simulink library "lib_controls"  (Simulink 7.9)
settings: Solver=ode45  SolverMode=SingleTasking  StartTime=0.0  StopTime=10.0  RelTol=1e-3
undefined symbols (not defined in the file or in its folder): amb_tmp, cs_charge_deplete_bool, cs_charge_pwr, cs_charge_trq, cs_clt_tmp, cs_decel_fc_off, cs_decel_regen_threshold, cs_dl_assist_trq_threshold, cs_dl_regen_trq_threshold, cs_electric_decel_spd, cs_electric_launch_spd, cs_electric_launch_spd_hi, cs_electric_launch_spd_lo, cs_eng_min_spd, cs_eng_on_soc, cs_fc_init_state, cs_fc_max_pwr_frac, cs_fc_min_pwr_frac, cs_fc_on, cs_fc_pwr_opt, cs_fc_spd_opt, cs_fuzzy_fuel_mode, cs_hi_soc, cs_hi_trq_frac, cs_lo_soc, cs_lo_trq_frac, cs_max_gc_spd, cs_max_pwr, cs_max_pwr_fall_rate, cs_max_pwr_rise_rate, cs_mc_assist_max_frac, cs_mc_assist_min_frac, cs_mc_assist_slope, cs_mc_regen_max_frac, cs_mc_regen_min_frac, cs_mc_regen_slope, cs_mean_eff, cs_mean_eff_bool, cs_min_gc_spd, cs_min_off_time, cs_min_pwr, cs_min_trq_frac, cs_mph_avg_time, cs_off_trq_frac, cs_plot_output, cs_pwr, cs_regen_avg_time, cs_scale_factor, cs_shutoff, cs_soc_range, cs_spd, cs_target_soc, cs_trq_to_soc_factor, cvt_locus_pwr, cvt_locus_spd, cyc_mph, enable_sim_stop_distance, enable_sim_stop_max_spd, enable_sim_stop_speed, enable_sim_stop_time ... (+110)
libraries: lib_controls x124, simulink3 x13, simulink x5, lib_etc x1
(part 10 of 17)

== system lib_controls/series hybrid control stategy  <cs>/pwr req'd from FC to supply pwr req'd at bus (W) ==
  power req'd by bus (W) : Inport
  Constant : Constant  Value=eps
  Constant1 : Constant  Value=eps
  Constant2 : Constant  Value=0
  Constant3 : Constant  Value=0
  Constant4 : Constant  Value=eps
  Relational Operator : RelationalOperator  Operator=>  InputSameDT=on
  Saturation : Saturate  UpperLimit=max(cs_pwr)  LowerLimit=min(cs_pwr)
  Sum : Sum  SaturateOnIntegerOverflow=on  InputSameDT=on  OutDataTypeStr=Inherit: Same as first input
  Sum1 : Sum  SaturateOnIntegerOverflow=on  InputSameDT=on  OutDataTypeStr=Inherit: Same as first input
  Sum2 : Sum  SaturateOnIntegerOverflow=on  InputSameDT=on  OutDataTypeStr=Inherit: Same as first input
  Switch : Switch  Threshold=eps  SaturateOnIntegerOverflow=on  InputSameDT=on
  est. efficiency : Product  Inputs=*/  SaturateOnIntegerOverflow=on  RndMeth=Zero  InputSameDT=on  OutDataTypeStr=Inherit: Same as first input
  est. desired spd (rad/s) : Lookup  InputValues=cs_pwr  Table=cs_spd  SaturateOnIntegerOverflow=on
  est. desired trq (Nm) : Product  Inputs=*/  SaturateOnIntegerOverflow=on  RndMeth=Zero  InputSameDT=on  OutDataTypeStr=Inherit: Same as first input
  est. pwr req'd into generator : Product  Inputs=/*  SaturateOnIntegerOverflow=on  RndMeth=Zero  InputSameDT=on  OutDataTypeStr=Inherit: Same as first input
  generator output power map (W) : Lookup2D  RowIndex=gc_map_spd*gc_spd_scale  ColumnIndex=gc_map_trq*gc_trq_scale  Table=gc_outpwr_map*gc_spd_scale*gc_trq_scale  SaturateOnIntegerOverflow=on  InputSameDT=on
  pwr req'd of FC (W) : Outport
  wires:
  power req'd by bus (W)/1 -> Relational Operator/1, Saturation/1
  Constant2/1 -> Relational Operator/2
  Constant1/1 -> Sum1/1
  Sum1/1 -> est. efficiency/2
  generator output power map (W)/1 -> est. efficiency/1
  Saturation/1 -> Sum1/2, est. pwr req'd into generator/2, est. desired trq (Nm)/1, est. desired spd (rad/s)/1
  est. desired spd (rad/s)/1 -> generator output power map (W)/1, Sum/1
  est. desired trq (Nm)/1 -> generator output power map (W)/2
  Constant/1 -> Sum/2
  Sum/1 -> est. desired trq (Nm)/2
  Constant3/1 -> Switch/3
  Relational Operator/1 -> Switch/2
  Switch/1 -> pwr req'd of FC (W)/1
  est. pwr req'd into generator/1 -> Switch/1
  est. efficiency/1 -> Sum2/1
  Sum2/1 -> est. pwr req'd into generator/1
  Constant4/1 -> Sum2/2

== system lib_controls/series hybrid control stategy  <cs>/thermostat ==

== system lib_controls/user contributed engine on (balanced parallel hybrid)/Block NOTES ==
  note: this user-contributed model came from Serve Ploumen-Research Engineer in Energy Management
      |  at Ford Forschungszentrum Aachen GmbH (Ford Research Centre Aachen)
      | The following is from the email:
      | For integrated Starter/generator equipped vehicles, we found it important to make the activation of
      | engine start-stop dependent on thetime needed for the engine-warmup (or catalyst warmup if you like)
      |  and also dependent in the SOC of the energy storage device. Furthermore we found
      | it important to delay the engine shut-down after the vehicle has come to a stop after a braking period.
      |
      | Therefore we implemented these functionality in the control strategy of Advisor's parallel hybrid model.

== system lib_controls/<vc> conv/clutch control/Block NOTES ==
  note: This clutch control block determines the clutch state given the req'd clutch output torque
      | and speed (labelled as gearbox input torque and speed), and the gear number history.
      |                           conditions                                                                       clutch state
      | gear is being shifted OR (trq <~ 0 AND (engine is                                     1 == disengaged
      | clutched to avoid compression braking OR spd < idle))
      |
      | (trq >~ 0) AND (spd < launch speed) AND clutch                                       2 == slipping
      | was not engaged during previous time step
      |
      | neither of above sets of conditions are met                                          3 == engaged

== system lib_controls/<vc> conv/clutch control/gearbox speed estimator ==
  gb_spd_in_r if no gear change : Inport
  Block NOTES : Subsystem
      mask Display: disp('Block\nNOTES')
  Constant : Constant  Value=eps
  Constant1 : Constant  Value=0
  Constant2 : Constant
  Constant3 : Constant  Value=0.11
  Gain : Gain  Gain=0.447  SaturateOnIntegerOverflow=on  OutDataTypeStr=Inherit: Same as input  ParamDataTypeStr=Inherit: Same as input
  Logical : Logic
  Memory : Memory  X0=cyc_mph(1,2)*0.447/wh_radius*fd_ratio*gb_ratio(gb_num_init)
  Memory1 : Memory  X0=1
  Product : Product  Inputs=**/  SaturateOnIntegerOverflow=on  RndMeth=Zero  InputSameDT=on  OutDataTypeStr=Inherit: Same as first input
  Relational : RelationalOperator  Operator=>  InputSameDT=on
  Relational1 : RelationalOperator  Operator=<=  InputSameDT=on
  Sum : Sum  SaturateOnIntegerOverflow=on  InputSameDT=on  OutDataTypeStr=Inherit: Same as first input
  Sum1 : Sum  Inputs=-+  SaturateOnIntegerOverflow=on  InputSameDT=on  OutDataTypeStr=Inherit: Same as first input
  Switch : Switch  Threshold=eps  SaturateOnIntegerOverflow=on  InputSameDT=on
  Switch1 : Switch  Threshold=eps  SaturateOnIntegerOverflow=on  InputSameDT=on
  dt : Subsystem
  Out1 : Outport
  wires:
  dt/1(Out1) -> Relational1/1
  Logical/1 -> Switch1/2
  Memory1/1 -> Logical/1
  Relational1/1 -> Logical/2
  Constant3/1 -> Relational1/2
  [gb_spd_in_a] -> Product/1
  gb_spd_in_r if no gear change/1 -> Switch1/3
  Switch1/1 -> Out1/1
  Switch/1 -> Memory/1
  Relational/1 -> Memory1/1
  Sum1/1 -> Relational/1
  Constant2/1 -> Relational/2
  [mpha] -> Sum1/1, Gain/1
  [cyc_mph_r] -> Sum1/2
  Constant/1 -> Sum/2
  Memory/1 -> Switch1/1
  Constant1/1 -> Switch/3
  [veh_spd_a_rec] -> Switch/2, Sum/1
  Gain/1 -> Product/2
  Sum/1 -> Product/3
  Product/1 -> Switch/1

== system lib_controls/<vc> conv/engine control/Block NOTES ==
  note: This engine control block determines whether the engine is on, which it is when
      | [(the clutch is slipping or engaged OR idling is allowed) AND the ignition key is on]
      | OR
      | (the transmission is shifting AND the engine was on during the previous time step).
      | The second part involving shifting is to prevent the engine from shutting down
      | for 1 or 2 seconds during shifts.

== system lib_controls/<vc> conv/engine control/key_on ==
  Clock : Clock
  Fcn1 : Fcn  Expr=rem(u[1],period)
  Look-Up Table : Lookup  InputValues=t  Table=y  SaturateOnIntegerOverflow=on
  out_1 : Outport  InitialOutput=0
  wires:
  Fcn1/1 -> Look-Up Table/1
  Clock/1 -> Fcn1/1
  Look-Up Table/1 -> out_1/1

== system lib_controls/<vc> conv/engine control/repeated cycle:  speed required at end of NEXT step ==
  Clock : Clock
  Fcn1 : Fcn  Expr=rem(u[1],period)
  Look-Up Table : Lookup  InputValues=t  Table=y  SaturateOnIntegerOverflow=on
  Memory : Memory  X0=-0.1
  Sum : Sum  Inputs=+-  SaturateOnIntegerOverflow=on  InputSameDT=on  OutDataTypeStr=Inherit: Same as first input
  Sum1 : Sum  SaturateOnIntegerOverflow=on  InputSameDT=on  OutDataTypeStr=Inherit: Same as first input
  out_1 : Outport  InitialOutput=0
  wires:
  Clock/1 -> Sum/1, Memory/1, Fcn1/1
  Memory/1 -> Sum/2
  Sum/1 -> Sum1/2
  Fcn1/1 -> Sum1/1
  Look-Up Table/1 -> out_1/1
  Sum1/1 -> Look-Up Table/1

== system lib_controls/<vc> conv/gearbox  control/Block NOTES ==
  note: This gearbox control block computes the current gear number given the gearbox's
      | req'd output torque and speed and an estimate its efficiency.  Upshifts occur, given a
      | certain engine speed,  when the estimated engine load falls below the upshift curve
      | in engine speed/load space, and downshifts likewise occur when estimated engine
      | load rises above the downshift curve.  Separate upshift and downshift curves are
      | defined for each gear.  An upshift may not be immediately followed by a downshift.
      | If the tires are about to slip, don't upshift unless the engine would be at max. speed.
      | Enforce this rule by setting the load to 1 when the tires are about to slip.

== system lib_controls/<vc> conv/gearbox  control/allow downshift? ==
  prev gearnum : Inport
  Logical Operator : Logic  Operator=NOR
  Memory : Memory  X0=1
  Memory1 : Memory  X0=1
  Relational Operator1 : RelationalOperator  Operator=>  InputSameDT=on
  Relational Operator2 : RelationalOperator  Operator=>  InputSameDT=on
  allow shift : Outport  InitialOutput=0
  wires:
  Relational Operator2/1 -> Logical Operator/2
  Memory1/1 -> Relational Operator2/2
  Memory/1 -> Memory1/1, Relational Operator1/2
  Relational Operator1/1 -> Logical Operator/1
  prev gearnum/1 -> Relational Operator2/1, Memory/1, Relational Operator1/1
  Logical Operator/1 -> allow shift/1

== system lib_controls/<vc> conv/gearbox  control/downshift  command ==
  prev gear number : Inport
  engine load : Inport  Port=2
  engine speed : Inport  Port=3
  Mux : Mux  Inputs=2
  Relational Operator : RelationalOperator  Operator=>  InputSameDT=on
  load fraction : Subsystem  mask(Gear Selector){spd=gb_dnshift_spd, load=gb_dnshift_load}
      mask prompts: spd "Speeds:"; load "Load Fractions:"
      mask help:
      | This block will perform a linear interplation (extrapolation outside of bounds) to determine the shift point load fraction associated with the current gear number and speed.
      |
      | The Speeds parameter should be defined as an array of vectors containing speeds for each gear number.  The Load Fractions parameter should be defined as a array of vectors containing load fractions indexed by the speeds in the Speeds parameter for each gear number.
      mask Help:
      | Reference the base workspace variables - gb_**shift_spd and gb_**shift_load  where ** is either up for upshift conditions or dn for downshift conditions.
      | 
      | Or define the arrays as follows:
      | 
      | {[spd1 spd2 spd3 spd4]; [spd1 spd2 spd3 spd4]; ...}
      | 
      | {[load1 load2 load3 load4]; [load1 load2 load3 load4]; ...}
      | 
      | where each array contains one row for each gear in the gearbox.  Speeds should be defined in rad/s and loads as a decimal fraction.
  command : Outport  InitialOutput=0
  wires:
  Relational Operator/1 -> command/1
  engine speed/1 -> Mux/2
  prev gear number/1 -> Mux/1
  engine load/1 -> Relational Operator/1
  Mux/1 -> load fraction/1(In1)
  load fraction/1(Out1) -> Relational Operator/2

== system lib_controls/<vc> conv/gearbox  control/gearbox speed estimator ==
  gb_spd_in_r if no gear change : Inport
  Block NOTES : Subsystem
      mask Display: disp('Block\nNOTES')
  Constant : Constant  Value=eps
  Constant1 : Constant  Value=0
  Constant2 : Constant
  Constant3 : Constant  Value=0.11
  Gain : Gain  Gain=0.447  SaturateOnIntegerOverflow=on  OutDataTypeStr=Inherit: Same as input  ParamDataTypeStr=Inherit: Same as input
  Logical : Logic
  Memory : Memory  X0=cyc_mph(1,2)*0.447/wh_radius*fd_ratio*gb_ratio(gb_num_init)
  Memory1 : Memory  X0=1
  Product : Product  Inputs=**/  SaturateOnIntegerOverflow=on  RndMeth=Zero  InputSameDT=on  OutDataTypeStr=Inherit: Same as first input
  Relational : RelationalOperator  Operator=>  InputSameDT=on
  Relational1 : RelationalOperator  Operator=<=  InputSameDT=on
  Sum : Sum  SaturateOnIntegerOverflow=on  InputSameDT=on  OutDataTypeStr=Inherit: Same as first input
  Sum1 : Sum  Inputs=-+  SaturateOnIntegerOverflow=on  InputSameDT=on  OutDataTypeStr=Inherit: Same as first input
  Switch : Switch  Threshold=eps  SaturateOnIntegerOverflow=on  InputSameDT=on
  Switch1 : Switch  Threshold=eps  SaturateOnIntegerOverflow=on  InputSameDT=on
  dt : Subsystem
  Out1 : Outport
  wires:
  dt/1(Out1) -> Relational1/1
  Logical/1 -> Switch1/2
  Memory1/1 -> Logical/1
  Relational1/1 -> Logical/2
  Constant3/1 -> Relational1/2
  [gb_spd_in_a] -> Product/1
  gb_spd_in_r if no gear change/1 -> Switch1/3
  Switch1/1 -> Out1/1
  Switch/1 -> Memory/1
  Relational/1 -> Memory1/1
  Sum1/1 -> Relational/1
  Constant2/1 -> Relational/2
  [mpha] -> Sum1/1, Gain/1
  [cyc_mph_r] -> Sum1/2
  Constant/1 -> Sum/2
  Memory/1 -> Switch1/1
  Constant1/1 -> Switch/3
  [veh_spd_a_rec] -> Switch/2, Sum/1
  Gain/1 -> Product/2
  Sum/1 -> Product/3
  Product/1 -> Switch/1

== system lib_controls/<vc> conv/gearbox  control/shifting1 ==
  gear number : Inport
  Constant : Constant  Value=gb_shift_delay-1e-6
  Relational Operator : RelationalOperator  Operator=<  InputSameDT=on
  time since last shift : Subsystem
      mask Display: disp('time since\nlast shift')
  out_1 : Outport  InitialOutput=0
  wires:
  time since last shift/1(out_1) -> Relational Operator/1
  Constant/1 -> Relational Operator/2
  gear number/1 -> time since last shift/1(in_1)
  Relational Operator/1 -> out_1/1

== system lib_controls/<vc> conv/gearbox  control/upshift  command ==
  prev gear number : Inport
  engine load : Inport  Port=2
  engine speed : Inport  Port=3
  Mux : Mux  Inputs=2
  Relational Operator : RelationalOperator  Operator=<  InputSameDT=on
  load fraction : Subsystem  mask(Gear Selector){spd=gb_upshift_spd, load=gb_upshift_load}
      mask prompts: spd "Speeds:"; load "Load Fractions:"
      mask help:
      | This block will perform a linear interplation (extrapolation outside of bounds) to determine the shift point load fraction associated with the current gear number and speed.
      |
      | The Speeds parameter should be defined as an array of vectors containing speeds for each gear number.  The Load Fractions parameter should be defined as a array of vectors containing load fractions indexed by the speeds in the Speeds parameter for each gear number.
      mask Help:
      | Reference the base workspace variables - gb_**shift_spd and gb_**shift_load  where ** is either up for upshift conditions or dn for downshift conditions.
      | 
      | Or define the arrays as follows:
      | 
      | {[spd1 spd2 spd3 spd4]; [spd1 spd2 spd3 spd4]; ...}
      | 
      | {[load1 load2 load3 load4]; [load1 load2 load3 load4]; ...}
      | 
      | where each array contains one row for each gear in the gearbox.  Speeds should be defined in rad/s and loads as a decimal fraction.
  command : Outport  InitialOutput=0
  wires:
  Relational Operator/1 -> command/1
  engine speed/1 -> Mux/2
  Mux/1 -> load fraction/1(In1)
  prev gear number/1 -> Mux/1
  engine load/1 -> Relational Operator/1
  load fraction/1(Out1) -> Relational Operator/2

== system lib_controls/<vc> conv Saber custom/clutch control/Block NOTES ==
  note: This clutch control block determines the clutch state given the req'd clutch output torque
      | and speed (labelled as gearbox input torque and speed), and the gear number history.
      |                           conditions                                                                       clutch state
      | gear is being shifted OR (trq <~ 0 AND (engine is                                     1 == disengaged
      | clutched to avoid compression braking OR spd < idle))
      |
      | (trq >~ 0) AND (spd < launch speed) AND clutch                                       2 == slipping
      | was not engaged during previous time step
      |
      | neither of above sets of conditions are met                                          3 == engaged

== system lib_controls/<vc> conv Saber custom/clutch control/gearbox speed estimator ==
  gb_spd_in_r if no gear change : Inport
  Block NOTES : Subsystem
      mask Display: disp('Block\nNOTES')
  Constant : Constant  Value=eps
  Constant1 : Constant  Value=0
  Constant2 : Constant
  Constant3 : Constant  Value=0.11
  Gain : Gain  Gain=0.447  SaturateOnIntegerOverflow=on  OutDataTypeStr=Inherit: Same as input  ParamDataTypeStr=Inherit: Same as input
  Logical : Logic
  Memory : Memory  X0=cyc_mph(1,2)*0.447/wh_radius*fd_ratio*gb_ratio(gb_num_init)
  Memory1 : Memory  X0=1
  Product : Product  Inputs=**/  SaturateOnIntegerOverflow=on  RndMeth=Zero  InputSameDT=on  OutDataTypeStr=Inherit: Same as first input
  Relational : RelationalOperator  Operator=>  InputSameDT=on
  Relational1 : RelationalOperator  Operator=<=  InputSameDT=on
  Sum : Sum  SaturateOnIntegerOverflow=on  InputSameDT=on  OutDataTypeStr=Inherit: Same as first input
  Sum1 : Sum  Inputs=-+  SaturateOnIntegerOverflow=on  InputSameDT=on  OutDataTypeStr=Inherit: Same as first input
  Switch : Switch  Threshold=eps  SaturateOnIntegerOverflow=on  InputSameDT=on
  Switch1 : Switch  Threshold=eps  SaturateOnIntegerOverflow=on  InputSameDT=on
  dt : Subsystem
  Out1 : Outport
  wires:
  Product/1 -> Switch/1
  Sum/1 -> Product/3
  Gain/1 -> Product/2
  [veh_spd_a_rec] -> Sum/1, Switch/2
  Constant1/1 -> Switch/3
  Memory/1 -> Switch1/1
  Constant/1 -> Sum/2
  [cyc_mph_r] -> Sum1/2
  [mpha] -> Gain/1, Sum1/1
  Constant2/1 -> Relational/2
  Sum1/1 -> Relational/1
  Relational/1 -> Memory1/1
  Switch/1 -> Memory/1
  Switch1/1 -> Out1/1
  gb_spd_in_r if no gear change/1 -> Switch1/3
  [gb_spd_in_a] -> Product/1
  Constant3/1 -> Relational1/2
  Relational1/1 -> Logical/2
  Memory1/1 -> Logical/1
  Logical/1 -> Switch1/2
  dt/1(Out1) -> Relational1/1

== system lib_controls/<vc> conv Saber custom/engine control/Block NOTES ==
  note: This engine control block determines whether the engine is on, which it is when
      | [(the clutch is slipping or engaged OR idling is allowed) AND the ignition key is on]
      | OR
      | (the transmission is shifting AND the engine was on during the previous time step).
      | The second part involving shifting is to prevent the engine from shutting down
      | for 1 or 2 seconds during shifts.

== system lib_controls/<vc> conv Saber custom/engine control/key_on ==
  Clock : Clock
  Fcn1 : Fcn  Expr=rem(u[1],period)
  Look-Up Table : Lookup  InputValues=t  Table=y  SaturateOnIntegerOverflow=on
  out_1 : Outport  InitialOutput=0
  wires:
  Look-Up Table/1 -> out_1/1
  Clock/1 -> Fcn1/1
  Fcn1/1 -> Look-Up Table/1

== system lib_controls/<vc> conv Saber custom/engine control/repeated cycle:  speed required at end of NEXT step ==
  Clock : Clock
  Fcn1 : Fcn  Expr=rem(u[1],period)
  Look-Up Table : Lookup  InputValues=t  Table=y  SaturateOnIntegerOverflow=on
  Memory : Memory  X0=-0.1
  Sum : Sum  Inputs=+-  SaturateOnIntegerOverflow=on  InputSameDT=on  OutDataTypeStr=Inherit: Same as first input
  Sum1 : Sum  SaturateOnIntegerOverflow=on  InputSameDT=on  OutDataTypeStr=Inherit: Same as first input
  out_1 : Outport  InitialOutput=0
  wires:
  Sum1/1 -> Look-Up Table/1
  Look-Up Table/1 -> out_1/1
  Fcn1/1 -> Sum1/1
  Sum/1 -> Sum1/2
  Memory/1 -> Sum/2
  Clock/1 -> Fcn1/1, Memory/1, Sum/1

== system lib_controls/<vc> conv Saber custom/gearbox  control/Block NOTES ==
  note: This gearbox control block computes the current gear number given the gearbox's
      | req'd output torque and speed and an estimate its efficiency.  Upshifts occur, given a
      | certain engine speed,  when the estimated engine load falls below the upshift curve
      | in engine speed/load space, and downshifts likewise occur when estimated engine
      | load rises above the downshift curve.  Separate upshift and downshift curves are
      | defined for each gear.  An upshift may not be immediately followed by a downshift.
      | If the tires are about to slip, don't upshift unless the engine would be at max. speed.
      | Enforce this rule by setting the load to 1 when the tires are about to slip.

== system lib_controls/<vc> conv Saber custom/gearbox  control/accessories (Nm) ==
  T_acc : Outport  InitialOutput=0
  wires:
  [fc_acc_trq_r] -> T_acc/1

== system lib_controls/<vc> conv Saber custom/gearbox  control/allow downshift? ==
  prev gearnum : Inport
  Logical Operator : Logic  Operator=NOR
  Memory : Memory  X0=1
  Memory1 : Memory  X0=1
  Relational Operator1 : RelationalOperator  Operator=>  InputSameDT=on
  Relational Operator2 : RelationalOperator  Operator=>  InputSameDT=on
  allow shift : Outport  InitialOutput=0
  wires:
  Logical Operator/1 -> allow shift/1
  prev gearnum/1 -> Relational Operator1/1, Memory/1, Relational Operator2/1
  Relational Operator1/1 -> Logical Operator/1
  Memory/1 -> Relational Operator1/2, Memory1/1
  Memory1/1 -> Relational Operator2/2
  Relational Operator2/1 -> Logical Operator/2

== system lib_controls/<vc> conv Saber custom/gearbox  control/downshift  command ==
  prev gear number : Inport
  engine load : Inport  Port=2
  engine speed : Inport  Port=3
  Mux : Mux  Inputs=2
  Relational Operator : RelationalOperator  Operator=>  InputSameDT=on
  load fraction : Subsystem  mask(Gear Selector){spd=gb_dnshift_spd, load=gb_dnshift_load}
      mask prompts: spd "Speeds:"; load "Load Fractions:"
      mask help:
      | This block will perform a linear interplation (extrapolation outside of bounds) to determine the shift point load fraction associated with the current gear number and speed.
      |
      | The Speeds parameter should be defined as an array of vectors containing speeds for each gear number.  The Load Fractions parameter should be defined as a array of vectors containing load fractions indexed by the speeds in the Speeds parameter for each gear number.
      mask Help:
      | Reference the base workspace variables - gb_**shift_spd and gb_**shift_load  where ** is either up for upshift conditions or dn for downshift conditions.
      | 
      | Or define the arrays as follows:
      | 
      | {[spd1 spd2 spd3 spd4]; [spd1 spd2 spd3 spd4]; ...}
      | 
      | {[load1 load2 load3 load4]; [load1 load2 load3 load4]; ...}
      | 
      | where each array contains one row for each gear in the gearbox.  Speeds should be defined in rad/s and loads as a decimal fraction.
  command : Outport  InitialOutput=0
  wires:
  load fraction/1(Out1) -> Relational Operator/2
  Mux/1 -> load fraction/1(In1)
  engine load/1 -> Relational Operator/1
  prev gear number/1 -> Mux/1
  engine speed/1 -> Mux/2
  Relational Operator/1 -> command/1

== system lib_controls/<vc> conv Saber custom/gearbox  control/gearbox speed estimator ==
  gb_spd_in_r if no gear change : Inport
  Block NOTES : Subsystem
      mask Display: disp('Block\nNOTES')
  Constant : Constant  Value=eps
  Constant1 : Constant  Value=0
  Constant2 : Constant
  Constant3 : Constant  Value=0.11
  Gain : Gain  Gain=0.447  SaturateOnIntegerOverflow=on  OutDataTypeStr=Inherit: Same as input  ParamDataTypeStr=Inherit: Same as input
  Logical : Logic
  Memory : Memory  X0=cyc_mph(1,2)*0.447/wh_radius*fd_ratio*gb_ratio(gb_num_init)
  Memory1 : Memory  X0=1
  Product : Product  Inputs=**/  SaturateOnIntegerOverflow=on  RndMeth=Zero  InputSameDT=on  OutDataTypeStr=Inherit: Same as first input
  Relational : RelationalOperator  Operator=>  InputSameDT=on
  Relational1 : RelationalOperator  Operator=<=  InputSameDT=on
  Sum : Sum  SaturateOnIntegerOverflow=on  InputSameDT=on  OutDataTypeStr=Inherit: Same as first input
  Sum1 : Sum  Inputs=-+  SaturateOnIntegerOverflow=on  InputSameDT=on  OutDataTypeStr=Inherit: Same as first input
  Switch : Switch  Threshold=eps  SaturateOnIntegerOverflow=on  InputSameDT=on
  Switch1 : Switch  Threshold=eps  SaturateOnIntegerOverflow=on  InputSameDT=on
  dt : Subsystem
  Out1 : Outport
  wires:
  Product/1 -> Switch/1
  Sum/1 -> Product/3
  Gain/1 -> Product/2
  [veh_spd_a_rec] -> Sum/1, Switch/2
  Constant1/1 -> Switch/3
  Memory/1 -> Switch1/1
  Constant/1 -> Sum/2
  [cyc_mph_r] -> Sum1/2
  [mpha] -> Gain/1, Sum1/1
  Constant2/1 -> Relational/2
  Sum1/1 -> Relational/1
  Relational/1 -> Memory1/1
  Switch/1 -> Memory/1
  Switch1/1 -> Out1/1
  gb_spd_in_r if no gear change/1 -> Switch1/3
  [gb_spd_in_a] -> Product/1
  Constant3/1 -> Relational1/2
  Relational1/1 -> Logical/2
  Memory1/1 -> Logical/1
  Logical/1 -> Switch1/2
  dt/1(Out1) -> Relational1/1

== system lib_controls/<vc> conv Saber custom/gearbox  control/shifting1 ==
  gear number : Inport
  Constant : Constant  Value=gb_shift_delay-1e-6
  Relational Operator : RelationalOperator  Operator=<  InputSameDT=on
  time since last shift : Subsystem
      mask Display: disp('time since\nlast shift')
  out_1 : Outport  InitialOutput=0
  wires:
  Relational Operator/1 -> out_1/1
  gear number/1 -> time since last shift/1(in_1)
  Constant/1 -> Relational Operator/2
  time since last shift/1(out_1) -> Relational Operator/1

== system lib_controls/<vc> conv Saber custom/gearbox  control/upshift  command ==
  prev gear number : Inport
  engine load : Inport  Port=2
  engine speed : Inport  Port=3
  Mux : Mux  Inputs=2
  Relational Operator : RelationalOperator  Operator=<  InputSameDT=on
  load fraction : Subsystem  mask(Gear Selector){spd=gb_upshift_spd, load=gb_upshift_load}
      mask prompts: spd "Speeds:"; load "Load Fractions:"
      mask help:
      | This block will perform a linear interplation (extrapolation outside of bounds) to determine the shift point load fraction associated with the current gear number and speed.
      |
      | The Speeds parameter should be defined as an array of vectors containing speeds for each gear number.  The Load Fractions parameter should be defined as a array of vectors containing load fractions indexed by the speeds in the Speeds parameter for each gear number.
      mask Help:
      | Reference the base workspace variables - gb_**shift_spd and gb_**shift_load  where ** is either up for upshift conditions or dn for downshift conditions.
      | 
      | Or define the arrays as follows:
      | 
      | {[spd1 spd2 spd3 spd4]; [spd1 spd2 spd3 spd4]; ...}
      | 
      | {[load1 load2 load3 load4]; [load1 load2 load3 load4]; ...}
      | 
      | where each array contains one row for each gear in the gearbox.  Speeds should be defined in rad/s and loads as a decimal fraction.
  command : Outport  InitialOutput=0
  wires:
  load fraction/1(Out1) -> Relational Operator/2
  engine load/1 -> Relational Operator/1
  prev gear number/1 -> Mux/1
  Mux/1 -> load fraction/1(In1)
  engine speed/1 -> Mux/2
  Relational Operator/1 -> command/1

== system lib_controls/<vc> conv auto/engine control/Block NOTES ==
  note: This engine control block determines whether the engine is on, which it is when
      | [(the clutch is slipping or engaged OR idling is allowed) AND the ignition key is on]
      | OR
      | (the transmission is shifting AND the engine was on during the previous time step).
      | The second part involving shifting is to prevent the engine from shutting down
      | for 1 or 2 seconds during shifts.

== system lib_controls/<vc> conv auto/engine control/key_on ==
  Clock : Clock
  Fcn1 : Fcn  Expr=rem(u[1],period)
  Look-Up Table : Lookup  InputValues=t  Table=y  SaturateOnIntegerOverflow=on
  out_1 : Outport  InitialOutput=0
  wires:
  Look-Up Table/1 -> out_1/1
  Clock/1 -> Fcn1/1
  Fcn1/1 -> Look-Up Table/1

== system lib_controls/<vc> conv auto/engine control/repeated cycle:  speed required at end of NEXT step ==
  Clock : Clock
  Fcn1 : Fcn  Expr=rem(u[1],period)
  Look-Up Table : Lookup  InputValues=t  Table=y  SaturateOnIntegerOverflow=on
  Memory : Memory  X0=-0.1
  Sum : Sum  Inputs=+-  SaturateOnIntegerOverflow=on  InputSameDT=on  OutDataTypeStr=Inherit: Same as first input
  Sum1 : Sum  SaturateOnIntegerOverflow=on  InputSameDT=on  OutDataTypeStr=Inherit: Same as first input
  out_1 : Outport  InitialOutput=0
  wires:
  Clock/1 -> Sum/1, Memory/1, Fcn1/1
  Memory/1 -> Sum/2
  Sum/1 -> Sum1/2
  Fcn1/1 -> Sum1/1
  Look-Up Table/1 -> out_1/1
  Sum1/1 -> Look-Up Table/1

== system lib_controls/<vc> conv auto/gearbox control for use w/ AT/Block NOTES ==
  note: This gearbox control block computes the current gear number given the gearbox's
      | req'd output torque and speed and an estimate its efficiency.  Upshifts occur, given a
      | certain engine speed,  when the estimated engine load falls below the upshift curve
      | in engine speed/load space, and downshifts likewise occur when estimated engine
      | load rises above the downshift curve.  Separate upshift and downshift curves are
      | defined for each gear.  An upshift may not be immediately followed by a downshift.
      | If the tires are about to slip, don't upshift unless the engine would be at max. speed.
      | Enforce this rule by setting the load to 1 when the tires are about to slip.
  note: Lock-up of the HTC occurs when it is supposed to for the current gear, AND
      | the transmission isn't shifting, AND
      | the lockup wouldn't precipitate an immediate downshift.

== system lib_controls/<vc> conv auto/gearbox control for use w/ AT/allow downshift? ==
  prev gearnum : Inport
  Logical Operator : Logic  Operator=NOR
  Memory : Memory  X0=1
  Memory1 : Memory  X0=1
  Relational Operator1 : RelationalOperator  Operator=>  InputSameDT=on
  Relational Operator2 : RelationalOperator  Operator=>  InputSameDT=on
  allow shift : Outport  InitialOutput=0
  wires:
  Relational Operator2/1 -> Logical Operator/2
  Memory1/1 -> Relational Operator2/2
  Memory/1 -> Memory1/1, Relational Operator1/2
  Relational Operator1/1 -> Logical Operator/1
  prev gearnum/1 -> Relational Operator2/1, Memory/1, Relational Operator1/1
  Logical Operator/1 -> allow shift/1

== system lib_controls/<vc> conv auto/gearbox control for use w/ AT/downshift  command ==
  prev gear number : Inport
  engine load : Inport  Port=2
  engine speed : Inport  Port=3
  Mux : Mux  Inputs=2
  Relational Operator : RelationalOperator  Operator=>  InputSameDT=on
  load fraction : Subsystem  mask(Gear Selector){spd=gb_dnshift_spd, load=gb_dnshift_load}
      mask prompts: spd "Speeds:"; load "Load Fractions:"
      mask help:
      | This block will perform a linear interplation (extrapolation outside of bounds) to determine the shift point load fraction associated with the current gear number and speed.
      |
      | The Speeds parameter should be defined as an array of vectors containing speeds for each gear number.  The Load Fractions parameter should be defined as a array of vectors containing load fractions indexed by the speeds in the Speeds parameter for each gear number.
      mask Help:
      | Reference the base workspace variables - gb_**shift_spd and gb_**shift_load  where ** is either up for upshift conditions or dn for downshift conditions.
      | 
      | Or define the arrays as follows:
      | 
      | {[spd1 spd2 spd3 spd4]; [spd1 spd2 spd3 spd4]; ...}
      | 
      | {[load1 load2 load3 load4]; [load1 load2 load3 load4]; ...}
      | 
      | where each array contains one row for each gear in the gearbox.  Speeds should be defined in rad/s and loads as a decimal fraction.
  command : Outport  InitialOutput=0
  wires:
  load fraction/1(Out1) -> Relational Operator/2
  Mux/1 -> load fraction/1(In1)
  engine load/1 -> Relational Operator/1
  prev gear number/1 -> Mux/1
  engine speed/1 -> Mux/2
  Relational Operator/1 -> command/1

== system lib_controls/<vc> conv auto/gearbox control for use w/ AT/downshift  command1 ==
  prev gear number : Inport
  engine load : Inport  Port=2
  engine speed : Inport  Port=3
  Mux : Mux  Inputs=2
  Relational Operator : RelationalOperator  Operator=>  InputSameDT=on
  load fraction : Subsystem  mask(Gear Selector){spd=gb_dnshift_spd, load=gb_dnshift_load}
      mask prompts: spd "Speeds:"; load "Load Fractions:"
      mask help:
      | This block will perform a linear interplation (extrapolation outside of bounds) to determine the shift point load fraction associated with the current gear number and speed.
      |
      | The Speeds parameter should be defined as an array of vectors containing speeds for each gear number.  The Load Fractions parameter should be defined as a array of vectors containing load fractions indexed by the speeds in the Speeds parameter for each gear number.
      mask Help:
      | Reference the base workspace variables - gb_**shift_spd and gb_**shift_load  where ** is either up for upshift conditions or dn for downshift conditions.
      | 
      | Or define the arrays as follows:
      | 
      | {[spd1 spd2 spd3 spd4]; [spd1 spd2 spd3 spd4]; ...}
      | 
      | {[load1 load2 load3 load4]; [load1 load2 load3 load4]; ...}
      | 
      | where each array contains one row for each gear in the gearbox.  Speeds should be defined in rad/s and loads as a decimal fraction.
  command : Outport  InitialOutput=0
  wires:
  Relational Operator/1 -> command/1
  prev gear number/1 -> Mux/1
  engine load/1 -> Relational Operator/1
  Mux/1 -> load fraction/1(In1)
  load fraction/1(Out1) -> Relational Operator/2
  engine speed/1 -> Mux/2

== system lib_controls/<vc> conv auto/gearbox control for use w/ AT/est. engine trq and spd ==
  prev gear number : Inport
  " prev eta_gb" : Inport  Port=2
  gb_trq_out_r : Inport  Port=3
  gb_spd_out_r : Inport  Port=4
  Block NOTES : Subsystem
      mask Display: disp('Block\nNOTES')
  Constant2 : Constant  Value=[1 1]
  Constant5 : Constant  Value=0
  Demux : Demux  Outputs=2
  K_adv : Subsystem
  Logical Operator : Logic
  Logical Operator1 : Logic  Operator=NOT  Inputs=1
  Memory : Memory
  Mux1 : Mux  Inputs=2
  Mux2 : Mux  Inputs=2
  Relational Operator1 : RelationalOperator  Operator=>  InputSameDT=on
  SR Look-Up Table SR=wout/win : Lookup  InputValues=htc_k_adv  Table=htc_sr  SaturateOnIntegerOverflow=on
  Saturation1 : Saturate  UpperLimit=1  LowerLimit=0.7
  Saturation2 : Saturate  UpperLimit=inf  LowerLimit=0
  Switch : Switch  Threshold=eps  SaturateOnIntegerOverflow=on  InputSameDT=on
  TR Look-Up Table TR=Tout/Tin : Lookup  InputValues=htc_k_adv  Table=htc_tr  SaturateOnIntegerOverflow=on
  TR,SR : Mux  Inputs=2
  est eng trq : Sum  SaturateOnIntegerOverflow=on  InputSameDT=on  OutDataTypeStr=Inherit: Same as first input
  gear ratio1 : Lookup  InputValues=[1:length(gb_ratio)]  Table=gb_ratio  SaturateOnIntegerOverflow=on
  ~eng trq and spd : Product  Inputs=*/  SaturateOnIntegerOverflow=on  RndMeth=Zero  InputSameDT=on  OutDataTypeStr=Inherit: Same as first input
  ~gb_spd_in_r : Product  SaturateOnIntegerOverflow=on  RndMeth=Zero  InputSameDT=on  OutDataTypeStr=Inherit: Same as first input
  ~gb_trq_in_r : Product  Inputs=//*  SaturateOnIntegerOverflow=on  RndMeth=Zero  InputSameDT=on  OutDataTypeStr=Inherit: Same as first input
  est eng trq (Nm) : Outport
  est eng spd (rad/s) : Outport  Port=2
  gb_spd_in_est (rad/s)1 : Outport  Port=3
  wires:
  gb_trq_out_r/1 -> ~gb_trq_in_r/3
  gb_spd_out_r/1 -> ~gb_spd_in_r/2
  gear ratio1/1 -> ~gb_trq_in_r/1, ~gb_spd_in_r/1
  TR,SR/1 -> Switch/1
  Constant2/1 -> Switch/3
  Switch/1 -> ~eng trq and spd/2
  " prev eta_gb"/1 -> Saturation1/1
  Saturation1/1 -> ~gb_trq_in_r/2
  Demux/2 -> Saturation2/1
  Saturation2/1 -> est eng spd (rad/s)/1
  Constant5/1 -> Relational Operator1/2
  Relational Operator1/1 -> Logical Operator/1
  prev gear number/1 -> gear ratio1/1
  Demux/1 -> est eng trq (Nm)/1
  Memory/1 -> Logical Operator1/1
  Logical Operator1/1 -> Logical Operator/2
  Logical Operator/1 -> Switch/2
  [locked_up] -> Memory/1
  Mux1/1 -> ~eng trq and spd/1
  ~eng trq and spd/1 -> Demux/1
  Mux2/1 -> K_adv/1("Req'd output trq and spd (Nm), (rad/s)")
  K_adv/1(K_adv) -> TR Look-Up Table TR=Tout/Tin/1, SR Look-Up Table SR=wout/win/1
  TR Look-Up Table TR=Tout/Tin/1 -> TR,SR/1
  SR Look-Up Table SR=wout/win/1 -> TR,SR/2
  [acc_mech_trq_est] -> est eng trq/2
  ~gb_spd_in_r/1 -> Mux1/2, gb_spd_in_est (rad/s)1/1, Mux2/2
  ~gb_trq_in_r/1 -> est eng trq/1
  est eng trq/1 -> Mux2/1, Relational Operator1/1, Mux1/1

== system lib_controls/<vc> conv auto/gearbox control for use w/ AT/est. engine trq and spd assuming lockup ==
  new gear number : Inport
  " prev eta_gb" : Inport  Port=2
  gb_trq_out_r : Inport  Port=3
  gb_spd_in_est : Inport  Port=4
  Block NOTES : Subsystem
      mask Display: disp('Block\nNOTES')
  Memory : Memory  X0=gb_ratio(1)
  Saturation1 : Saturate  UpperLimit=1  LowerLimit=0.7
  Saturation2 : Saturate  UpperLimit=inf  LowerLimit=0
  est eng trq : Sum  SaturateOnIntegerOverflow=on  InputSameDT=on  OutDataTypeStr=Inherit: Same as first input
  gear ratio1 : Lookup  InputValues=[1:length(gb_ratio)]  Table=gb_ratio  SaturateOnIntegerOverflow=on
  ~gb_spd_in_r : Product  Inputs=*/*  SaturateOnIntegerOverflow=on  RndMeth=Zero  InputSameDT=on  OutDataTypeStr=Inherit: Same as first input
  ~gb_trq_in_r : Product  Inputs=//*  SaturateOnIntegerOverflow=on  RndMeth=Zero  InputSameDT=on  OutDataTypeStr=Inherit: Same as first input
  est eng trq (Nm) : Outport
  est eng spd (rad/s) : Outport  Port=2
  wires:
  Saturation1/1 -> ~gb_trq_in_r/2
  " prev eta_gb"/1 -> Saturation1/1
  gear ratio1/1 -> ~gb_trq_in_r/1, ~gb_spd_in_r/1, Memory/1
  gb_trq_out_r/1 -> ~gb_trq_in_r/3
  new gear number/1 -> gear ratio1/1
  Saturation2/1 -> est eng spd (rad/s)/1
  Memory/1 -> ~gb_spd_in_r/2
  gb_spd_in_est/1 -> ~gb_spd_in_r/3
  [acc_mech_trq_est] -> est eng trq/2
  ~gb_trq_in_r/1 -> est eng trq/1
  est eng trq/1 -> est eng trq (Nm)/1
  ~gb_spd_in_r/1 -> Saturation2/1

== system lib_controls/<vc> conv auto/gearbox control for use w/ AT/shifting1 ==
  gear number : Inport
  Constant : Constant  Value=gb_shift_delay-1e-6
  Relational Operator : RelationalOperator  Operator=<  InputSameDT=on
  time since last shift : Subsystem
      mask Display: disp('time since\nlast shift')
  out_1 : Outport  InitialOutput=0
  wires:
  time since last shift/1(out_1) -> Relational Operator/1
  Constant/1 -> Relational Operator/2
  gear number/1 -> time since last shift/1(in_1)
  Relational Operator/1 -> out_1/1

== system lib_controls/<vc> conv auto/gearbox control for use w/ AT/upshift  command ==
  prev gear number : Inport
  engine load : Inport  Port=2
  engine speed : Inport  Port=3
  Mux : Mux  Inputs=2
  Relational Operator : RelationalOperator  Operator=<  InputSameDT=on
  load fraction : Subsystem  mask(Gear Selector){spd=gb_upshift_spd, load=gb_upshift_load}
      mask prompts: spd "Speeds:"; load "Load Fractions:"
      mask help:
      | This block will perform a linear interplation (extrapolation outside of bounds) to determine the shift point load fraction associated with the current gear number and speed.
      |
      | The Speeds parameter should be defined as an array of vectors containing speeds for each gear number.  The Load Fractions parameter should be defined as a array of vectors containing load fractions indexed by the speeds in the Speeds parameter for each gear number.
      mask Help:
      | Reference the base workspace variables - gb_**shift_spd and gb_**shift_load  where ** is either up for upshift conditions or dn for downshift conditions.
      | 
      | Or define the arrays as follows:
      | 
      | {[spd1 spd2 spd3 spd4]; [spd1 spd2 spd3 spd4]; ...}
      | 
      | {[load1 load2 load3 load4]; [load1 load2 load3 load4]; ...}
      | 
      | where each array contains one row for each gear in the gearbox.  Speeds should be defined in rad/s and loads as a decimal fraction.
  command : Outport  InitialOutput=0
  wires:
  load fraction/1(Out1) -> Relational Operator/2
  engine load/1 -> Relational Operator/1
  prev gear number/1 -> Mux/1
  Mux/1 -> load fraction/1(In1)
  engine speed/1 -> Mux/2
  Relational Operator/1 -> command/1

== system lib_controls/<vc> conv auto Saber custom/engine control/Block NOTES ==
  note: This engine control block determines whether the engine is on, which it is when
      | [(the clutch is slipping or engaged OR idling is allowed) AND the ignition key is on]
      | OR
      | (the transmission is shifting AND the engine was on during the previous time step).
      | The second part involving shifting is to prevent the engine from shutting down
      | for 1 or 2 seconds during shifts.

== system lib_controls/<vc> conv auto Saber custom/engine control/key_on ==
  Clock : Clock
  Fcn1 : Fcn  Expr=rem(u[1],period)
  Look-Up Table : Lookup  InputValues=t  Table=y  SaturateOnIntegerOverflow=on
  out_1 : Outport  InitialOutput=0
  wires:
  Fcn1/1 -> Look-Up Table/1
  Clock/1 -> Fcn1/1
  Look-Up Table/1 -> out_1/1

== system lib_controls/<vc> conv auto Saber custom/engine control/repeated cycle:  speed required at end of NEXT step ==
  Clock : Clock
  Fcn1 : Fcn  Expr=rem(u[1],period)
  Look-Up Table : Lookup  InputValues=t  Table=y  SaturateOnIntegerOverflow=on
  Memory : Memory  X0=-0.1
  Sum : Sum  Inputs=+-  SaturateOnIntegerOverflow=on  InputSameDT=on  OutDataTypeStr=Inherit: Same as first input
  Sum1 : Sum  SaturateOnIntegerOverflow=on  InputSameDT=on  OutDataTypeStr=Inherit: Same as first input
  out_1 : Outport  InitialOutput=0
  wires:
  Sum1/1 -> Look-Up Table/1
  Look-Up Table/1 -> out_1/1
  Fcn1/1 -> Sum1/1
  Sum/1 -> Sum1/2
  Memory/1 -> Sum/2
  Clock/1 -> Fcn1/1, Memory/1, Sum/1

== system lib_controls/<vc> conv auto Saber custom/gearbox control for use w/ AT/Block NOTES ==
  note: Lock-up of the HTC occurs when it is supposed to for the current gear, AND
      | the transmission isn't shifting, AND
      | the lockup wouldn't precipitate an immediate downshift.
  note: This gearbox control block computes the current gear number given the gearbox's
      | req'd output torque and speed and an estimate its efficiency.  Upshifts occur, given a
      | certain engine speed,  when the estimated engine load falls below the upshift curve
      | in engine speed/load space, and downshifts likewise occur when estimated engine
      | load rises above the downshift curve.  Separate upshift and downshift curves are
      | defined for each gear.  An upshift may not be immediately followed by a downshift.
      | If the tires are about to slip, don't upshift unless the engine would be at max. speed.
      | Enforce this rule by setting the load to 1 when the tires are about to slip.

== system lib_controls/<vc> conv auto Saber custom/gearbox control for use w/ AT/allow downshift? ==
  prev gearnum : Inport
  Logical Operator : Logic  Operator=NOR
  Memory : Memory  X0=1
  Memory1 : Memory  X0=1
  Relational Operator1 : RelationalOperator  Operator=>  InputSameDT=on
  Relational Operator2 : RelationalOperator  Operator=>  InputSameDT=on
  allow shift : Outport  InitialOutput=0
  wires:
  Logical Operator/1 -> allow shift/1
  prev gearnum/1 -> Relational Operator1/1, Memory/1, Relational Operator2/1
  Relational Operator1/1 -> Logical Operator/1
  Memory/1 -> Relational Operator1/2, Memory1/1
  Memory1/1 -> Relational Operator2/2
  Relational Operator2/1 -> Logical Operator/2

== system lib_controls/<vc> conv auto Saber custom/gearbox control for use w/ AT/downshift  command ==
  prev gear number : Inport
  engine load : Inport  Port=2
  engine speed : Inport  Port=3
  Mux : Mux  Inputs=2
  Relational Operator : RelationalOperator  Operator=>  InputSameDT=on
  load fraction : Subsystem  mask(Gear Selector){spd=gb_dnshift_spd, load=gb_dnshift_load}
      mask prompts: spd "Speeds:"; load "Load Fractions:"
      mask help:
      | This block will perform a linear interplation (extrapolation outside of bounds) to determine the shift point load fraction associated with the current gear number and speed.
      |
      | The Speeds parameter should be defined as an array of vectors containing speeds for each gear number.  The Load Fractions parameter should be defined as a array of vectors containing load fractions indexed by the speeds in the Speeds parameter for each gear number.
      mask Help:
      | Reference the base workspace variables - gb_**shift_spd and gb_**shift_load  where ** is either up for upshift conditions or dn for downshift conditions.
      | 
      | Or define the arrays as follows:
      | 
      | {[spd1 spd2 spd3 spd4]; [spd1 spd2 spd3 spd4]; ...}
      | 
      | {[load1 load2 load3 load4]; [load1 load2 load3 load4]; ...}
      | 
      | where each array contains one row for each gear in the gearbox.  Speeds should be defined in rad/s and loads as a decimal fraction.
  command : Outport  InitialOutput=0
  wires:
  Relational Operator/1 -> command/1
  engine speed/1 -> Mux/2
  prev gear number/1 -> Mux/1
  engine load/1 -> Relational Operator/1
  Mux/1 -> load fraction/1(In1)
  load fraction/1(Out1) -> Relational Operator/2

== system lib_controls/<vc> conv auto Saber custom/gearbox control for use w/ AT/downshift  command1 ==
  prev gear number : Inport
  engine load : Inport  Port=2
  engine speed : Inport  Port=3
  Mux : Mux  Inputs=2
  Relational Operator : RelationalOperator  Operator=>  InputSameDT=on
  load fraction : Subsystem  mask(Gear Selector){spd=gb_dnshift_spd, load=gb_dnshift_load}
      mask prompts: spd "Speeds:"; load "Load Fractions:"
      mask help:
      | This block will perform a linear interplation (extrapolation outside of bounds) to determine the shift point load fraction associated with the current gear number and speed.
      |
      | The Speeds parameter should be defined as an array of vectors containing speeds for each gear number.  The Load Fractions parameter should be defined as a array of vectors containing load fractions indexed by the speeds in the Speeds parameter for each gear number.
      mask Help:
      | Reference the base workspace variables - gb_**shift_spd and gb_**shift_load  where ** is either up for upshift conditions or dn for downshift conditions.
      | 
      | Or define the arrays as follows:
      | 
      | {[spd1 spd2 spd3 spd4]; [spd1 spd2 spd3 spd4]; ...}
      | 
      | {[load1 load2 load3 load4]; [load1 load2 load3 load4]; ...}
      | 
      | where each array contains one row for each gear in the gearbox.  Speeds should be defined in rad/s and loads as a decimal fraction.
  command : Outport  InitialOutput=0
  wires:
  engine speed/1 -> Mux/2
  load fraction/1(Out1) -> Relational Operator/2
  Mux/1 -> load fraction/1(In1)
  engine load/1 -> Relational Operator/1
  prev gear number/1 -> Mux/1
  Relational Operator/1 -> command/1

== system lib_controls/<vc> conv auto Saber custom/gearbox control for use w/ AT/est. engine trq and spd ==
  prev gear number : Inport
  " prev eta_gb" : Inport  Port=2
  gb_trq_out_r : Inport  Port=3
  gb_spd_out_r : Inport  Port=4
  Block NOTES : Subsystem
      mask Display: disp('Block\nNOTES')
  Constant2 : Constant  Value=[1 1]
  Constant5 : Constant  Value=0
  Demux : Demux  Outputs=2
  K_adv : Subsystem
  Logical Operator : Logic
  Logical Operator1 : Logic  Operator=NOT  Inputs=1
  Memory : Memory
  Mux1 : Mux  Inputs=2
  Mux2 : Mux  Inputs=2
  Relational Operator1 : RelationalOperator  Operator=>  InputSameDT=on
  SR Look-Up Table SR=wout/win : Lookup  InputValues=htc_k_adv  Table=htc_sr  SaturateOnIntegerOverflow=on
  Saturation1 : Saturate  UpperLimit=1  LowerLimit=0.7
  Saturation2 : Saturate  UpperLimit=inf  LowerLimit=0
  Switch : Switch  Threshold=eps  SaturateOnIntegerOverflow=on  InputSameDT=on
  TR Look-Up Table TR=Tout/Tin : Lookup  InputValues=htc_k_adv  Table=htc_tr  SaturateOnIntegerOverflow=on
  TR,SR : Mux  Inputs=2
  accessories (Nm) : Subsystem
  est eng trq : Sum  SaturateOnIntegerOverflow=on  InputSameDT=on  OutDataTypeStr=Inherit: Same as first input
  gear ratio1 : Lookup  InputValues=[1:length(gb_ratio)]  Table=gb_ratio  SaturateOnIntegerOverflow=on
  ~eng trq and spd : Product  Inputs=*/  SaturateOnIntegerOverflow=on  RndMeth=Zero  InputSameDT=on  OutDataTypeStr=Inherit: Same as first input
  ~gb_spd_in_r : Product  SaturateOnIntegerOverflow=on  RndMeth=Zero  InputSameDT=on  OutDataTypeStr=Inherit: Same as first input
  ~gb_trq_in_r : Product  Inputs=//*  SaturateOnIntegerOverflow=on  RndMeth=Zero  InputSameDT=on  OutDataTypeStr=Inherit: Same as first input
  est eng trq (Nm) : Outport
  est eng spd (rad/s) : Outport  Port=2
  gb_spd_in_est (rad/s)1 : Outport  Port=3
  wires:
  est eng trq/1 -> Mux1/1, Relational Operator1/1, Mux2/1
  ~gb_trq_in_r/1 -> est eng trq/1
  accessories (Nm)/1(Out1) -> est eng trq/2
  SR Look-Up Table SR=wout/win/1 -> TR,SR/2
  TR Look-Up Table TR=Tout/Tin/1 -> TR,SR/1
  K_adv/1(K_adv) -> SR Look-Up Table SR=wout/win/1, TR Look-Up Table TR=Tout/Tin/1
  Mux2/1 -> K_adv/1("Req'd output trq and spd (Nm), (rad/s)")
  ~eng trq and spd/1 -> Demux/1
  Mux1/1 -> ~eng trq and spd/1
  [locked_up] -> Memory/1
  Logical Operator/1 -> Switch/2
  Logical Operator1/1 -> Logical Operator/2
  Memory/1 -> Logical Operator1/1
  Demux/1 -> est eng trq (Nm)/1
  prev gear number/1 -> gear ratio1/1
  Relational Operator1/1 -> Logical Operator/1
  Constant5/1 -> Relational Operator1/2
  Saturation2/1 -> est eng spd (rad/s)/1
  Demux/2 -> Saturation2/1
  Saturation1/1 -> ~gb_trq_in_r/2
  " prev eta_gb"/1 -> Saturation1/1
  Switch/1 -> ~eng trq and spd/2
  Constant2/1 -> Switch/3
  TR,SR/1 -> Switch/1
  gear ratio1/1 -> ~gb_spd_in_r/1, ~gb_trq_in_r/1
  gb_spd_out_r/1 -> ~gb_spd_in_r/2
  gb_trq_out_r/1 -> ~gb_trq_in_r/3
  ~gb_spd_in_r/1 -> Mux2/2, gb_spd_in_est (rad/s)1/1, Mux1/2
